simulink model "AdaptiveCruiseControl_HapticInterface"  (R2022b)
settings: Solver=FixedStepDiscrete  StartTime=0.0  StopTime=10.0  FixedStep=0.0005  RelTol=1e-3  EnableMultiTasking=on
InitFcn:
  | mbd_s32k_consistency_checks(bdroot(gcs));
values from neighbouring files (symbols this model uses):
  Ak = 100    [parameters_template.m]
  b = 100    [parameters_template.m]
  base_ids = [10, 0, 0, 0, 0, 0]    [parameters_template.m]
  dT = 0.01    [parameters_template.m]
  H = 20    [parameters_template.m]
  Kd = 0.0358    [parameters_template.m]
  Kdm = 137.4    [parameters_template.m]
  Kp = 0.256    [parameters_template.m]
  Kpm = 573.45    [parameters_template.m]
  L1 = 1.6    [parameters_template.m]
  L2 = 0.8    [parameters_template.m]
  m = 2000    [parameters_template.m]
  n_desired = 0    [parameters_template.m]
  pot_gain = 0.8    [parameters_template.m]
  pot_offset = 512    [parameters_template.m]
  R = 1/5    (= 0.2)    [parameters_template.m]
  V_Ki = 50    [parameters_template.m]
  V_Kp = 5000    [parameters_template.m]
undefined symbols (not defined in the file or in its folder): DiscIntNeverNeededParam, LQFP
libraries: mbd_s32k1xx_ec_toolbox x38, slrealtimeutilitieslib x15, Veh_Sim x9, simulink x3
(part 1 of 2)
settings Model: Creator=raoulkumar  LastModifiedBy=jyotshna
settings SolverCC: AlgebraicLoopSolver=TrustRegion  AutoInsertRateTranBlk=on
settings DataIOCC: ExternalInput=off  InitialState=off  LimitDataPoints=on  SaveOutput=off  SignalLogging=off  SaveTime=off  ReturnWorkspaceOutputs=off
settings OptimizationCC: DefaultParameterBehavior=Inlined  UseDivisionForNetSlopeComputation=on  UseFloatMulNetSlope=on  InlineInvariantSignals=on  EnhancedBackFolding=on  PassReuseOutputArgsAs=Individual arguments  ZeroExternalMemoryAtStartup=off  ZeroInternalMemoryAtStartup=off  NoFixptDivByZeroProtection=on  EfficientFloat2IntCast=on  OptimizeBlockOrder=speed  DifferentSizesBufferReuse=on  OptimizationCustomize=off  EfficientTunableParamExpr=on
settings DebuggingCC: InheritedTsInSrcMsg=none  SingleTaskRateTransMsg=error  ParameterTunabilityLossMsg=error  UnconnectedInputMsg=error  UnconnectedOutputMsg=error  UnconnectedLineMsg=error  AllowSymbolicDim=off  UnknownTsInhSupMsg=error  SFUnexpectedBacktrackingDiag=warning  SFNoUnconditionalDefaultTransitionDiag=warning  SFExecutionAtInitializationDiag=none  SFMachineParentedDataDiag=warning  ArithmeticOperatorsInVariantConditions=warning
settings HardwareCC: ProdBitPerPointer=32  ProdBitPerSizeT=32  ProdBitPerPtrDiffT=32  ProdLargestAtomicInteger=Long  ProdLargestAtomicFloat=Double  ProdWordSize=32  ProdHWDeviceType=ARM Compatible->ARM Cortex
settings ModelReferenceCC: EnableRefExpFcnMdlSchedulingChecks=on  PropagateSignalLabelsOutOfModel=off
settings SFSimCC: SimUseLocalCustomCode=off  MATLABDynamicMemAlloc=off  CustomCodeUndefinedFunction=UseInterfaceOnly
settings RTWCC: Description=Model Based Design Toolbox S32K1xx Code Generation Target  SystemTargetFile=mbd_s32k.tlc  MakeCommand=mbd_s32k_make_rtw COPY_MDLREF_INCLUDES=0  TemplateMakefile=mbd_s32k.tmf  GenerateReport=on  RTWUseLocalCustomCode=off  CustomHeaderCode=#include <math.h>  CustomSource=path_data.c;  IncludeHyperlinkInReport=on  LaunchReport=on  GenerateTraceInfo=on  GenerateTraceReport=on  GenerateTraceReportSl=on  GenerateTraceReportSf=on  GenerateTraceReportEml=on  GenerateCodeMetricsReport=on  DLArmComputeVersion=19.05
settings CodeAppCC: ForceParamTrailComments=on  IgnoreCustomStorageClasses=off  OperatorAnnotations=on  SimulinkDataObjDesc=on  SFDataObjDesc=on  CustomSymbolStrGlobalVar=rt$N$M  CustomSymbolStrType=$N$M  CustomSymbolStrFcn=$N$M$F  CustomSymbolStrMacro=$N$M  InsertBlockDesc=on
settings STFCustomTargetCC: TargetLangStandard=C99 (ISO)  MultiwordLength=256  CombineOutputUpdateFcns=on  ERTCustomFileBanners=on  SupportContinuousTime=off  SupportNonInlinedSFcns=off  RemoveResetFunc=on  MATLABClassNameForMDSCustomization=Simulink.SoftwareTarget.ERTCustomization  SystemTargetFile=mbd_s32k.tlc
settings ERTTargetCC: TargetLangStandard=C99 (ISO)  ParMdlRefBuildCompliant=off  CompOptLevelCompliant=off  ConcurrentExecutionCompliant=off  ModelStepFunctionPrototypeControlCompliant=off  CPPClassGenCompliant=off  UseToolchainInfoCompliant=off  InlinedParameterPlacement=NonHierarchical  ERTSrcFileBannerTemplate=mbd_ert_code_template.cgt  ERTHdrFileBannerTemplate=mbd_ert_code_template.cgt  ERTDataSrcFileTemplate=mbd_ert_code_template.cgt  ERTDataHdrFileTemplate=mbd_ert_code_template.cgt  ERTCustomFileTemplate=example_file_process.tlc
settings ConfigComp: CovMetricSettings=dw  CovSaveCumulativeToWorkspaceVar=on  CovSaveSingleToWorkspaceVar=on  CovExternalEMLEnable=off

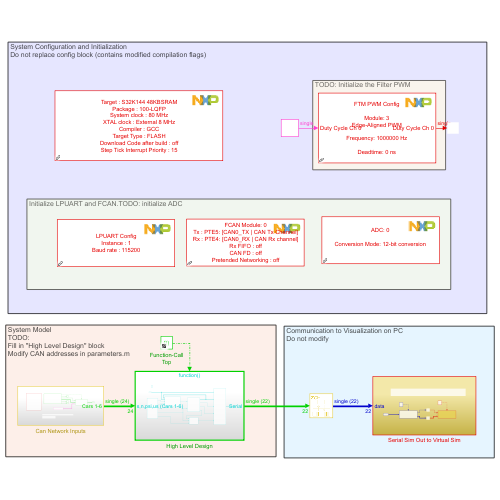
[thumbnail: Simulink's stored preview of the top-level diagram]
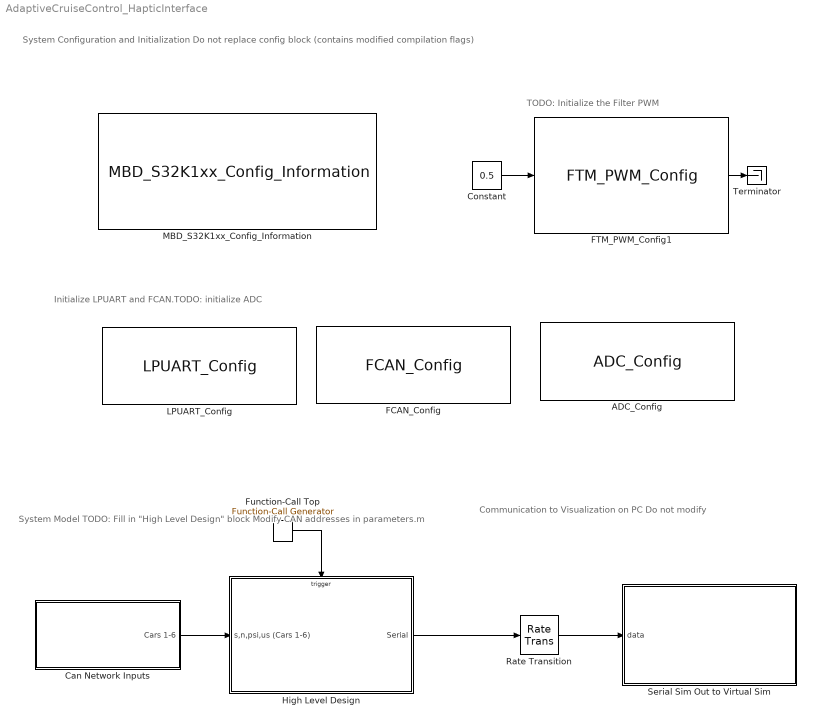
== system AdaptiveCruiseControl_HapticInterface ==
  note: TODO: Initialize the Filter PWM
  note: Communication to Visualization on PC
      | Do not modify
  note: Initialize LPUART and FCAN.TODO: initialize ADC
  note: System Configuration and Initialization
      | Do not replace config block (contains modified compilation flags)
  note: System Model
      | TODO:
      | Fill in "High Level Design" block
      | Modify CAN addresses in parameters.m
  ADC_Config : mbd_s32k1xx_ec_toolbox/Motor Control Blocks/ADC Blocks/ADC_Config  instance=0  mode=12-bit conversion  smplts=2  adiclk=alternate clock 1  adiv=input clock  show_adv_opts=off  pretrgsel=PDB pre-trigger  swpretrg=Disabled  adtrg=software  trgsel=TRGMUX output  refsel=Vrefh and Vrefl  supply_monitoring=off  acfe=off  acfgt=off  acren=off  cv1=0  cv2=0  adco=off  avge=off  avgs=4 samples
  Can Network Inputs : Subsystem
  Constant : Constant  Value=0.5  OutDataTypeStr=single
  FCAN_Config : mbd_s32k1xx_ec_toolbox/Communication Blocks/CAN Blocks/FCAN_Config  Priority=2  can_instance=0  can_mode=Normal mode  can_max_num_mb=32  can_rx=PTE4: [CAN0_RX | CAN Rx channel]  can_tx=PTE5: [CAN0_TX | CAN Tx Channel]  show_adv_opts=on  can_clk_src=Peripheral clock  can_clk_freq=80 MHz  bitrate_to_time_seg=on  bitrate=500  sample_point=80  real_bitrate=500  real_sample_point=80  prop_delay=250  bus_length=1  tq=200.0  time_quanta=10  can_presdiv=16  can_propseg=3  can_pseg1=4  can_pseg2=2  can_rjw=2  cbt_bitrate=2000  cbt_sample_point=80  cbt_real_bitrate=2000  cbt_real_sample_point=80  cbt_tq=25.0  cbt_time_quanta=40  can_cbt_presdiv=3  can_cbt_propseg=6  can_cbt_pseg1=7  can_cbt_pseg2=7  can_cbt_rjw=3  can_fd_enable=off  can_payload=8  tdc_enable=off  tdc_offset=20  can_rxfifo_enable=off  can_num_id_filters=8  can_fifo_id_format=A  can_fifo_id_filter={'0x0', '0x0', '0x0', '0x0', '0x0', '0x0', '0x0', '0x0'}  can_pn_enable=off  can_wakeup_match=off  can_wakeup_timeout=off  can_timeout_en=off  can_match_timeout=1  can_multiple_matches_en=off  can_num_matches=1  can_idfilter_extendedid=off  can_idfilter_remoteframe=off  can_idfilter_type=Match exact  can_idfilter_id1=0  can_idfilter_id2=0  can_payloadfilter_enable=off  can_payloadfilter_dlclow=0  can_payloadfilter_dlchigh=0  can_payloadfilter_type=Match exact  can_payloadfilter_payload1_b0=0  can_payloadfilter_payload1_b1=0  can_payloadfilter_payload1_b2=0  can_payloadfilter_payload1_b3=0  can_payloadfilter_payload1_b4=0  can_payloadfilter_payload1_b5=0  can_payloadfilter_payload1_b6=0  can_payloadfilter_payload1_b7=0  can_payloadfilter_payload2_b0=0  can_payloadfilter_payload2_b1=0  can_payloadfilter_payload2_b2=0  can_payloadfilter_payload2_b3=0  can_payloadfilter_payload2_b4=0  can_payloadfilter_payload2_b5=0  can_payloadfilter_payload2_b6=0  can_payloadfilter_payload2_b7=0
  FTM_PWM_Config1 : mbd_s32k1xx_ec_toolbox/Motor Control Blocks/FTM Blocks/FTM_PWM_Config  ftmModule=3  ftmMode=Edge-Aligned PWM  ftmSourceClock=80 MHz  swcontrol_enable=off  chan0En=on  chan0Type=Complementary  chan2En=off  chan2Type=Independent  chan4En=off  chan4Type=Independent  chan6En=off  chan6Type=Independent  ftmPwmUnits=Hz  outFrequency=1000000  ftmPeriod=80  ftmPrescaler=Divide by 1  deadtimeUnits=Nanoseconds  deadtimeNs=0  deadtimeTicks=0  deadtimePrescaler=Divide by 1  dutyCycleCh0=0.25  dutyCycleCh1=0.25  dutyCycleCh2=0.25  dutyCycleCh3=0.25  dutyCycleCh4=0.25  dutyCycleCh5=0.25  dutyCycleCh6=0.25  dutyCycleCh7=0.25  dutyCycleSim=on  startAfterInit=on  showAdvOpt=on  pinFtmCh0=PTB8: [FTM3_CH0 | FTM Channel]  pinFtmCh1=None  pinPolCh0=Active High  pinPolCh1=Active Low  outputComplem0=Main duplicated  outputLevel0=Low  outputLevel1=Low  pinFtmCh2=PTB10: [FTM3_CH2 | FTM Channel]  pinFtmCh3=None  pinPolCh2=Active Low  pinPolCh3=Active Low  outputComplem2=Main duplicated  outputLevel2=Low  outputLevel3=Low  pinFtmCh4=PTC10: [FTM3_CH4 | FTM Channel]  pinFtmCh5=None  pinPolCh4=Active Low  pinPolCh5=Active Low  outputComplem4=Main duplicated  outputLevel4=Low  outputLevel5=Low  pinFtmCh6=PTC12: [FTM3_CH6 | FTM Channel]  pinFtmCh7=None  pinPolCh6=Active Low  pinPolCh7=Active Low  outputComplem6=Main duplicated  outputLevel6=Low  outputLevel7=Low  initTrigger=off  chTrigger0=off  chTrigger1=off  chTrigger2=off  chTrigger3=off  chTrigger4=off  chTrigger5=off  chTrigger6=off  chTrigger7=off  mcuTargetUpdate=on  pwmSyncTrg=Software trigger  pwmSyncHwRouting=TRGMUX_FTM7  pwmSyncTrg0=off  pwmSyncTrg1=off  pwmSyncTrg2=off  pwmSyncAutoClear=on  pwmSyncMinLoad=on  pwmSyncMaxLoad=on  pwmSyncInvert=System Clock  pwmSyncOutControl=System Clock  pwmSyncOutMask=System Clock  pwmSyncCounterInitial=System Clock  pwmSyncPoints=Update now  reloadEnable=off  reloadPriority=15  reloadHalfCycle=off  reloadHCR=0  reloadFrequency=0  chnMatch0=off  chnMatch1=off  chnMatch2=off  chnMatch3=off  chnMatch4=off  chnMatch5=off  chnMatch6=off  chnMatch7=off  pwmFaultProtection=off  pwmFaultInterrupt=off  pwmFaultClearing=Fault control disabled  pwmFaultPinState=Safe Value  pwmFaultFilterValue=0  pwmFaultPriority=15  fault_disen_0=off  fault_filter_0=off  fault_polarity_0=Active High  fault_disen_1=off  fault_filter_1=off  fault_polarity_1=Active high  fault_disen_2=off  fault_filter_2=off  fault_polarity_2=Active high  fault_disen_3=off  fault_filter_3=off  fault_polarity_3=Active high  fault_pin_0=None  fault_pin_1=None  fault_pin_2=None  fault_pin_3=None
  Function-Call Top : simulink/Ports & Subsystems/Function-Call Generator  sample_time=dT  numberOfIterations=1  DisallowWideOutput=off
  High Level Design : Subsystem  TreatAsAtomicUnit=on
  LPUART_Config : mbd_s32k1xx_ec_toolbox/Communication Blocks/UART Blocks/LPUART_Config  Priority=2  instance=1  baudrate=115200  custom_baudrate=1000000  databits=8  parity=None  sbns=1  bothedge=rising edge  rxinv=off  txinv=off  show_adv_opts=on  brk13=10 - 13 bit times  lbkde=10 - 13 bit times  rx=PTC6: [LPUART1_RX | Receive]  tx=PTC7: [LPUART1_TX | Transmit]
  MBD_S32K1xx_Config_Information : mbd_s32k1xx_ec_toolbox/MBD_S32K1xx_Config_Information  mbdt_ver=0  disp_str=|  config_params=[]  mcu_target_name=S32K144  mcu_target_package=100-LQFP  mcu_target_sram_size=48KB  mcu_system_clock_freq=80  mcu_xtal_freq=External 8  mcu_steptick_timer=LPIT Channel 0  mcu_steptick_prio=15  ds_import_enable=on  target_compiler=GCC  target_memory=FLASH  gcc_target_compile_opts=-mthumb -mfloat-abi=hard -mfpu=fpv4-sp-d16 -O1 -g -gstrict-dwarf -DRT -DmwSize=size_t -include stdbool.h  gcc_target_assemble_opts=-mthumb -mfloat-abi=hard -mfpu=fpv4-sp-d16 -g  gcc_target_link_opts=-mthumb -mfloat-abi=hard -mfpu=fpv4-sp-d16  gcc_target_default_lcf=on  gcc_target_user_lcf=S32K144_48_flash.ld  ghs_target_compile_opts=-cpu=cortexm4f -thumb -fpu=vfpv4_d16 -fsingle -Ogeneral -Wundef -Wimplicit-int -Wshadow -Wtrigraphs --no_commons --gnu_asm -gnu99 -gdwarf-2 -G  ghs_target_assemble_opts=-cpu=cortexm4f -fpu=vfpv4_d16  ghs_target_link_opts=-cpu=cortexm4f -thumb -fpu=vfpv4_d16  ghs_target_default_lcf=on  ghs_target_user_lcf=S32K144_48_flash.ld  iar_target_compile_opts=--cpu=Cortex-M4F --thumb --fpu=VFPv4_sp -Ol -e --debug --dlib_config normal  iar_target_assemble_opts=--cpu Cortex-M4F --thumb --fpu VFPv4_sp  iar_target_link_opts=--no_exceptions --vfe --inline  iar_target_default_lcf=on  iar_target_user_lcf=S32K144_48_flash.icf  pil_download_enable=off  rbl_download_enable=off  rbl_start_delay=5000  rbl_download_interface=OpenSDA  rbl_restart_request=off  rbl_com_port=Custom  rbl_com_port_custom=COM1  pil_download_rate=57600  pil_download_rate_custom=115200  pil_opensda_drive=E: EVB-S32K144  pil_opensda_drive_custom=D  jtag_interface=OpenSDA Embedded Debug  jlink_default_path=on  jlink_user_path=C:\Program Files\SEGGER\JLink\  pil_uart_instance=1  pil_uart_rx=PTC6: [LPUART1_RX | Receive]  pil_uart_tx=PTC7: [LPUART1_TX | Transmit]  FTM_PWM_PcrCheckEnDis=on  FTM_Input_Edge_Inputs_PcrCheckEnDis=on  FTM_Dual_Edge_Inputs_PcrCheckEnDis=on  FTM_Quadrature_Inputs_PcrCheckEnDis=on  FTM_Hall_Sensor_Inputs_PcrCheckEnDis=on  LPTMR_PcrCheckEnDis=on  PIT_PcrCheckEnDis=on  RTC_PcrCheckEnDis=on  FlexCAN_PcrCheckEnDis=on  LIN_PcrCheckEnDis=on  FlexIO_PcrCheckEnDis=on  LPI2C_PcrCheckEnDis=on  LPSPI_PcrCheckEnDis=on  LPUART_PcrCheckEnDis=on  CMP_PcrCheckEnDis=on  GPIO_OutputPcrCheckEnDis=on  GPIO_InputPcrCheckEnDis=on  SBC_PcrCheckEnDis=on  BMS_PcrCheckEnDis=on  AMMCLIB_PcrCheckEnDis=on  FM_PcrCheckEnDis=on  Profile_PcrCheckEnDis=on  ConfigParams_PcrCheckEnDis=on  ModelRef_PcrCheckEnDis=on  PDB0_PcrCheckEnDis=on  CSEc_PcrCheckEnDis=on  eDMA_PcrCheckEnDis=on  FLASH_PcrCheckEnDis=on  ADC_PcrCheckEnDis=on  WDOG_PcrCheckEnDis=on
      | Target : S32K144-64KB_SRAM
      | Package : 100-pin
      | System clock : 80 MHz
      | XTAL clock : External 8 MHz
      | Compiler : IAR
      | Target Type : FLASH
      | Download Code after build : off
      | Step Tick Interrupt Priority : 15
  Rate Transition : RateTransition
  Serial Sim Out to Virtual Sim : Subsystem
  Terminator : Terminator
  wires:
  High Level Design/1(Serial) -> Rate Transition/1
  Function-Call Top/1 -> High Level Design/Trigger
  Rate Transition/1 -> Serial Sim Out to Virtual Sim/1(data)
  Can Network Inputs/1(Cars 1-6) -> High Level Design/1(s,n,psi,us (Cars 1-6))
  Constant/1 -> FTM_PWM_Config1/1
  FTM_PWM_Config1/1 -> Terminator/1

== system AdaptiveCruiseControl_HapticInterface/Can Network Inputs ==
  note: Do not modify anything here
      | Set base IDs in the parameters file
  note: These blocks may not display properly until CAN configuration has been comleted
  Array of 6 base IDs : Constant  Value=base_ids
  Can Message Mailbox Setup : Subsystem
  Extract CAN data : Subsystem
  FCAN_Isr : mbd_s32k1xx_ec_toolbox/Communication Blocks/CAN Blocks/FCAN_Isr  can_instance=0  can_event=Rx Complete
  Terminator1 : Terminator
  Terminator2 : Terminator
  Terminator3 : Terminator
  Cars 1-6 : Outport  VectorParamsAs1DForOutWhenUnconnected=off
  wires:
  FCAN_Isr/5 -> Terminator1/1
  Array of 6 base IDs/1 -> Extract CAN data/3(CAN Base IDs (Cars 1-6))
  FCAN_Isr/4 -> Extract CAN data/2(data)
  FCAN_Isr/6 -> Terminator3/1
  FCAN_Isr/1 -> Extract CAN data/Trigger
  Extract CAN data/1("s, n, psi, us (Cars 1-6)") -> Cars 1-6/1
  FCAN_Isr/2 -> Terminator2/1
  FCAN_Isr/3 -> Extract CAN data/1(ID)

== system AdaptiveCruiseControl_HapticInterface/High Level Design ==
  s,n,psi,us (Cars 1-6) : Inport
  function : TriggerPort  TriggerType=function-call  VariantControl=(inherit)
  ACC : Subsystem
  Auto Steer : Subsystem
  Inputs : Subsystem
  Outputs : Subsystem
  Vehicle Dynamics : Subsystem
  Serial : Outport  VectorParamsAs1DForOutWhenUnconnected=off
  wires:
  Outputs/1("x, y, pxi (Cars 1-6)") -> Serial/1
  Inputs/4(Steering Angle (delta)) -> Vehicle Dynamics/2(delta), Auto Steer/2(delta)
  Vehicle Dynamics/3(self-align torque) -> Outputs/4(Self-Aligning Torque)
  Vehicle Dynamics/2(u (this car)) -> Outputs/3(u (This car))
  Vehicle Dynamics/1(s,n,psi,u_s (this car)) -> ACC/1(s,n,psi,us (This car)), Outputs/2("s, n, psi, us (This Car)")
  s,n,psi,us (Cars 1-6)/1 -> ACC/2(s,n,psi,us (Cars 1-6)), Outputs/1("s, n, psi, us (Cars 1-6)")
  Inputs/1(ACC_enable) -> ACC/3(ACC_EN)
  Inputs/2(Cruise Control Speed) -> ACC/4(Cruise Speed)
  Inputs/3(Throttle (Fd)) -> ACC/5(Throttle)
  ACC/1(F_d) -> Vehicle Dynamics/1(F_d)
  Auto Steer/1(Auto Torque) -> Outputs/5(Auto Torque)
  Vehicle Dynamics/4(n) -> Auto Steer/1(n)
  Inputs/5(Automatic Steering Enable) -> Auto Steer/3(AS_EN)

== system AdaptiveCruiseControl_HapticInterface/Serial Sim Out to Virtual Sim ==
  note: UART transmission is non-blocking.
      | We must wait for transmission to complete before sending the next byte.
      | Could use LPUART interrupts block or just periodcally transmit to allow time for buffer to clear
  data : Inport
  Function-Call Generator1 : simulink/Ports & Subsystems/Function-Call Generator  sample_time=0.05  numberOfIterations=1  DisallowWideOutput=off
  Function-Call Generator2 : simulink/Ports & Subsystems/Function-Call Generator  sample_time=0.05 / 100  numberOfIterations=1  DisallowWideOutput=off
  RT : RateTransition  OutPortSampleTimeOpt=Inherit  OutPortSampleTime=0.0005
  RT1 : RateTransition  OutPortSampleTimeOpt=Inherit  OutPortSampleTime=0.0005
  Serial : Subsystem  TreatAsAtomicUnit=on
  UART Iteration : Subsystem
  wires:
  Serial/1(reset) -> RT/1
  Serial/2(data_out) -> RT1/1
  data/1 -> Serial/1(data)
  Function-Call Generator1/1 -> Serial/Trigger
  RT/1 -> UART Iteration/1(reset)
  Function-Call Generator2/1 -> UART Iteration/Trigger
  RT1/1 -> UART Iteration/2(data)

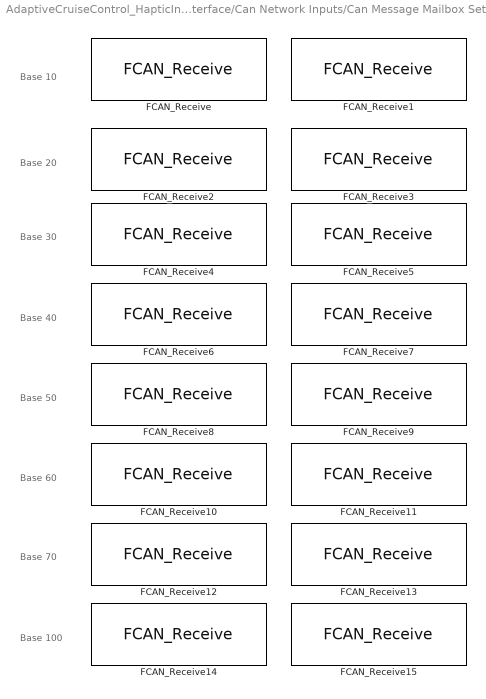
== system AdaptiveCruiseControl_HapticInterface/Can Network Inputs/Can Message Mailbox Setup ==
  note: Base 10
  note: Base 20
  note: Base 30
  note: Base 40
  note: Base 50
  note: Base 60
  note: Base 70
  note: Base 100
  FCAN_Receive : mbd_s32k1xx_ec_toolbox/Communication Blocks/CAN Blocks/FCAN_Receive  can_instance=0  can_mode=Non-blocking  can_timeout_ms=0  can_mb_idx=16  can_mb_init=Once  show_id_input=off  can_extended_id=off  can_is_remote=off  can_id=0F  can_msg_mask=0  show_adv_opts=on  can_use_rxfifo=off  can_fd_enable=off
  FCAN_Receive1 : mbd_s32k1xx_ec_toolbox/Communication Blocks/CAN Blocks/FCAN_Receive  can_instance=0  can_mode=Non-blocking  can_timeout_ms=0  can_mb_idx=17  can_mb_init=Once  show_id_input=off  can_extended_id=off  can_is_remote=off  can_id=10  can_msg_mask=0  show_adv_opts=on  can_use_rxfifo=off  can_fd_enable=off
  FCAN_Receive10 : mbd_s32k1xx_ec_toolbox/Communication Blocks/CAN Blocks/FCAN_Receive  can_instance=0  can_mode=Non-blocking  can_timeout_ms=0  can_mb_idx=12  can_mb_init=Once  show_id_input=off  can_extended_id=off  can_is_remote=off  can_id=41  can_msg_mask=0  show_adv_opts=on  can_use_rxfifo=off  can_fd_enable=off
  FCAN_Receive11 : mbd_s32k1xx_ec_toolbox/Communication Blocks/CAN Blocks/FCAN_Receive  can_instance=0  can_mode=Non-blocking  can_timeout_ms=0  can_mb_idx=13  can_mb_init=Once  show_id_input=off  can_extended_id=off  can_is_remote=off  can_id=42  can_msg_mask=0  show_adv_opts=on  can_use_rxfifo=off  can_fd_enable=off
  FCAN_Receive12 : mbd_s32k1xx_ec_toolbox/Communication Blocks/CAN Blocks/FCAN_Receive  can_instance=0  can_mode=Non-blocking  can_timeout_ms=0  can_mb_idx=2  can_mb_init=Once  show_id_input=off  can_extended_id=off  can_is_remote=off  can_id=4b  can_msg_mask=0  show_adv_opts=on  can_use_rxfifo=off  can_fd_enable=off
  FCAN_Receive13 : mbd_s32k1xx_ec_toolbox/Communication Blocks/CAN Blocks/FCAN_Receive  can_instance=0  can_mode=Non-blocking  can_timeout_ms=0  can_mb_idx=3  can_mb_init=Once  show_id_input=off  can_extended_id=off  can_is_remote=off  can_id=4c  can_msg_mask=0  show_adv_opts=on  can_use_rxfifo=off  can_fd_enable=off
  FCAN_Receive14 : mbd_s32k1xx_ec_toolbox/Communication Blocks/CAN Blocks/FCAN_Receive  can_instance=0  can_mode=Non-blocking  can_timeout_ms=0  can_mb_idx=14  can_mb_init=Once  show_id_input=off  can_extended_id=off  can_is_remote=off  can_id=69  can_msg_mask=0  show_adv_opts=on  can_use_rxfifo=off  can_fd_enable=off
  FCAN_Receive15 : mbd_s32k1xx_ec_toolbox/Communication Blocks/CAN Blocks/FCAN_Receive  can_instance=0  can_mode=Non-blocking  can_timeout_ms=0  can_mb_idx=15  can_mb_init=Once  show_id_input=off  can_extended_id=off  can_is_remote=off  can_id=6a  can_msg_mask=0  show_adv_opts=on  can_use_rxfifo=off  can_fd_enable=off
  FCAN_Receive2 : mbd_s32k1xx_ec_toolbox/Communication Blocks/CAN Blocks/FCAN_Receive  can_instance=0  can_mode=Non-blocking  can_timeout_ms=0  can_mb_idx=4  can_mb_init=Once  show_id_input=off  can_extended_id=off  can_is_remote=off  can_id=19  can_msg_mask=0  show_adv_opts=on  can_use_rxfifo=off  can_fd_enable=off
  FCAN_Receive3 : mbd_s32k1xx_ec_toolbox/Communication Blocks/CAN Blocks/FCAN_Receive  can_instance=0  can_mode=Non-blocking  can_timeout_ms=0  can_mb_idx=5  can_mb_init=Once  show_id_input=off  can_extended_id=off  can_is_remote=off  can_id=1a  can_msg_mask=0  show_adv_opts=on  can_use_rxfifo=off  can_fd_enable=off
  FCAN_Receive4 : mbd_s32k1xx_ec_toolbox/Communication Blocks/CAN Blocks/FCAN_Receive  can_instance=0  can_mode=Non-blocking  can_timeout_ms=0  can_mb_idx=6  can_mb_init=Once  show_id_input=off  can_extended_id=off  can_is_remote=off  can_id=23  can_msg_mask=0  show_adv_opts=on  can_use_rxfifo=off  can_fd_enable=off
  FCAN_Receive5 : mbd_s32k1xx_ec_toolbox/Communication Blocks/CAN Blocks/FCAN_Receive  can_instance=0  can_mode=Non-blocking  can_timeout_ms=0  can_mb_idx=7  can_mb_init=Once  show_id_input=off  can_extended_id=off  can_is_remote=off  can_id=24  can_msg_mask=0  show_adv_opts=on  can_use_rxfifo=off  can_fd_enable=off
  FCAN_Receive6 : mbd_s32k1xx_ec_toolbox/Communication Blocks/CAN Blocks/FCAN_Receive  can_instance=0  can_mode=Non-blocking  can_timeout_ms=0  can_mb_idx=8  can_mb_init=Once  show_id_input=off  can_extended_id=off  can_is_remote=off  can_id=2d  can_msg_mask=0  show_adv_opts=on  can_use_rxfifo=off  can_fd_enable=off
  FCAN_Receive7 : mbd_s32k1xx_ec_toolbox/Communication Blocks/CAN Blocks/FCAN_Receive  can_instance=0  can_mode=Non-blocking  can_timeout_ms=0  can_mb_idx=9  can_mb_init=Once  show_id_input=off  can_extended_id=off  can_is_remote=off  can_id=2e  can_msg_mask=0  show_adv_opts=on  can_use_rxfifo=off  can_fd_enable=off
  FCAN_Receive8 : mbd_s32k1xx_ec_toolbox/Communication Blocks/CAN Blocks/FCAN_Receive  can_instance=0  can_mode=Non-blocking  can_timeout_ms=0  can_mb_idx=10  can_mb_init=Once  show_id_input=off  can_extended_id=off  can_is_remote=off  can_id=37  can_msg_mask=0  show_adv_opts=on  can_use_rxfifo=off  can_fd_enable=off
  FCAN_Receive9 : mbd_s32k1xx_ec_toolbox/Communication Blocks/CAN Blocks/FCAN_Receive  can_instance=0  can_mode=Non-blocking  can_timeout_ms=0  can_mb_idx=11  can_mb_init=Once  show_id_input=off  can_extended_id=off  can_is_remote=off  can_id=38  can_msg_mask=0  show_adv_opts=on  can_use_rxfifo=off  can_fd_enable=off

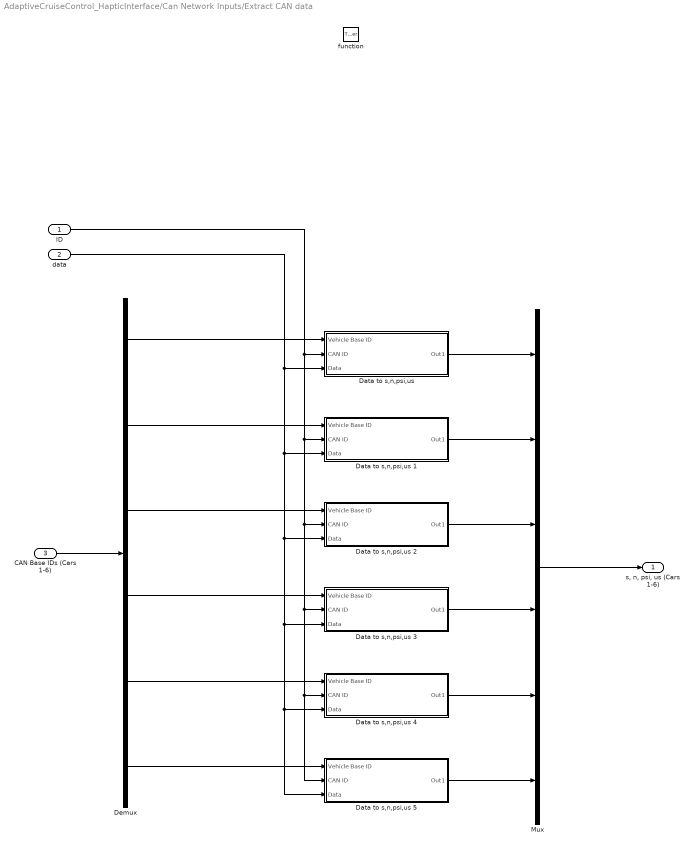
== system AdaptiveCruiseControl_HapticInterface/Can Network Inputs/Extract CAN data ==
  ID : Inport
  data : Inport  Port=2
  CAN Base IDs (Cars 1-6) : Inport  Port=3
  function : TriggerPort  TriggerType=function-call  VariantControl=Variant
  "Data to s,n,psi,us " : Subsystem
  Data to s,n,psi,us 1 : Subsystem
  Data to s,n,psi,us 2 : Subsystem
  Data to s,n,psi,us 3 : Subsystem
  Data to s,n,psi,us 4 : Subsystem
  Data to s,n,psi,us 5 : Subsystem
  Demux : Demux  Outputs=6
  Mux : Mux  Inputs=6
  "s, n, psi, us (Cars 1-6)" : Outport  VectorParamsAs1DForOutWhenUnconnected=off
  wires:
  Mux/1 -> "s, n, psi, us (Cars 1-6)"/1
  ID/1 -> Data to s,n,psi,us 5/2(CAN ID), Data to s,n,psi,us 4/2(CAN ID), Data to s,n,psi,us 3/2(CAN ID), Data to s,n,psi,us 2/2(CAN ID), Data to s,n,psi,us 1/2(CAN ID), "Data to s,n,psi,us "/2(CAN ID)
  "Data to s,n,psi,us "/1(Out1) -> Mux/1
  Data to s,n,psi,us 1/1(Out1) -> Mux/2
  Data to s,n,psi,us 2/1(Out1) -> Mux/3
  Data to s,n,psi,us 3/1(Out1) -> Mux/4
  Data to s,n,psi,us 4/1(Out1) -> Mux/5
  Data to s,n,psi,us 5/1(Out1) -> Mux/6
  data/1 -> Data to s,n,psi,us 5/3(Data), Data to s,n,psi,us 4/3(Data), Data to s,n,psi,us 3/3(Data), Data to s,n,psi,us 2/3(Data), Data to s,n,psi,us 1/3(Data), "Data to s,n,psi,us "/3(Data)
  Demux/1 -> "Data to s,n,psi,us "/1(Vehicle Base ID)
  Demux/2 -> Data to s,n,psi,us 1/1(Vehicle Base ID)
  Demux/3 -> Data to s,n,psi,us 2/1(Vehicle Base ID)
  Demux/4 -> Data to s,n,psi,us 3/1(Vehicle Base ID)
  Demux/5 -> Data to s,n,psi,us 4/1(Vehicle Base ID)
  Demux/6 -> Data to s,n,psi,us 5/1(Vehicle Base ID)
  CAN Base IDs (Cars 1-6)/1 -> Demux/1

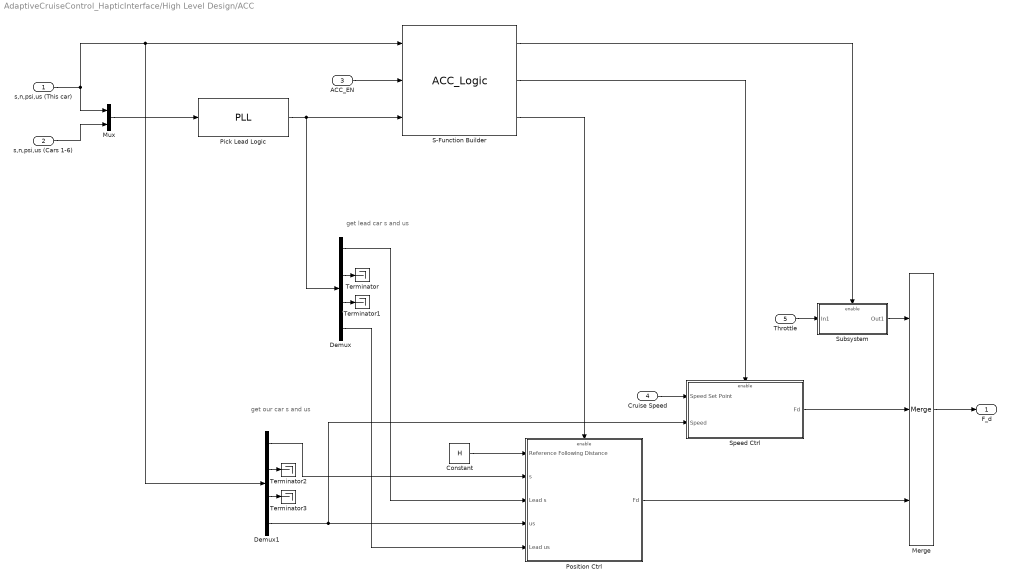
== system AdaptiveCruiseControl_HapticInterface/High Level Design/ACC ==
  note: get our car s and us
  note: get lead car s and us
  s,n,psi,us (This car) : Inport
  s,n,psi,us (Cars 1-6) : Inport  Port=2
  ACC_EN : Inport  Port=3
  Cruise Speed : Inport  Port=4
  Throttle : Inport  Port=5
  Constant : Constant  Value=H
  Demux : Demux
  Demux1 : Demux
  Merge : Merge  Inputs=3
  Mux : Mux  Inputs=2
  Pick Lead Logic : S-Function  FunctionName=PLL  SFunctionModules=PLL_wrapper.c  SFunctionDeploymentMode=off  EnableBusSupport=off  mask(S-Function Builder){}
      mask help: Simulink:masks:SFunctionBuilder_MD
      mask init:
      | val = [[.9  0.75 0.75 1 1 .9 .9 1]',[1 1 0.75 0.75 .9 .9 1 .9]'];try , sys = get_param(gcb,'SfunBuilderFcnName');if isempty(sys), sys = get_param(gcb,'FunctionName'); end,catch, sys = get_param(gcb,'FunctionName'); end
      settings: CopyFcn=set_param(gcbh,'LinkStatus','none')  OpenFcn=sfunctionwizard(gcbh)
      mask Display:
      | plot(val(:,1),val(:,2))
      | disp(sys)
      | port_label('input',1,'cars')
      | port_label('output',1,'lead')
  Position Ctrl : Subsystem  TreatAsAtomicUnit=on
  S-Function Builder : S-Function  FunctionName=ACC_Logic  Parameters=single(H)  SFunctionModules=ACC_Logic_wrapper.c  SFunctionDeploymentMode=off  EnableBusSupport=off  mask(S-Function Builder){}
      mask help: Simulink:masks:SFunctionBuilder_MD
      mask init: same as AdaptiveCruiseControl_HapticInterface/High Level Design/ACC/Pick Lead Logic
      settings: CopyFcn=set_param(gcbh,'LinkStatus','none')  OpenFcn=sfunctionwizard(gcbh)
      mask Display:
      | plot(val(:,1),val(:,2))
      | disp(sys)
      | port_label('input',1,'our_car')
      | port_label('input',2,'ACC_EN')
      | port_label('input',3,'lead_car')
      | port_label('output',1,'MAN_EN')
      | port_label('output',2,'VEL_EN')
      | port_label('output',3,'POS_EN')
  Speed Ctrl : Subsystem  TreatAsAtomicUnit=on
  Subsystem : Subsystem
  Terminator{,1..3} (4 alike) : Terminator
  F_d : Outport
  wires:
  S-Function Builder/1 -> Subsystem/Enable
  Demux/1 -> Position Ctrl/3(Lead s)
  Demux/3 -> Terminator1/1
  Demux1/2 -> Terminator2/1
  s,n,psi,us (This car)/1 -> Mux/1, Demux1/1, S-Function Builder/1
  s,n,psi,us (Cars 1-6)/1 -> Mux/2
  Demux1/1 -> Position Ctrl/2(s)
  Mux/1 -> Pick Lead Logic/1
  ACC_EN/1 -> S-Function Builder/2
  Position Ctrl/1(Fd) -> Merge/3
  Demux/4 -> Position Ctrl/5(Lead us)
  S-Function Builder/3 -> Position Ctrl/Enable
  Subsystem/1(Out1) -> Merge/1
  Pick Lead Logic/1 -> Demux/1, S-Function Builder/3
  Constant/1 -> Position Ctrl/1(Reference Following Distance)
  Throttle/1 -> Subsystem/1(In1)
  Demux/2 -> Terminator/1
  Demux1/4 -> Speed Ctrl/2(Speed), Position Ctrl/4(us)
  Demux1/3 -> Terminator3/1
  Cruise Speed/1 -> Speed Ctrl/1(Speed Set Point)
  Speed Ctrl/1(Fd) -> Merge/2
  S-Function Builder/2 -> Speed Ctrl/Enable
  Merge/1 -> F_d/1

== system AdaptiveCruiseControl_HapticInterface/High Level Design/Auto Steer ==
  n : Inport
  delta : Inport  Port=2
  AS_EN : Inport  Port=3
  S-Function Builder1 : S-Function  Commented=on  FunctionName=auto_steer  Parameters=single(n_desired),single(Kp),single(Kd),single(Kpm),single(Kdm)  SFunctionModules=auto_steer_wrapper.c  SFunctionDeploymentMode=off  EnableBusSupport=off  mask(S-Function Builder){}
      mask help: Simulink:masks:SFunctionBuilder_MD
      mask init: same as AdaptiveCruiseControl_HapticInterface/High Level Design/ACC/Pick Lead Logic
      settings: CopyFcn=set_param(gcbh,'LinkStatus','none')  OpenFcn=sfunctionwizard(gcbh)
      mask Display:
      | plot(val(:,1),val(:,2))
      | disp(sys)
      | port_label('input',1,'n')
      | port_label('input',2,'delta')
      | port_label('input',3,'AS_EN')
      | port_label('output',1,'t_auto')
  Subsystem1 : Subsystem
  Auto Torque : Outport
  wires:
  n/1 -> Subsystem1/1(n)
  delta/1 -> Subsystem1/2(delta)
  AS_EN/1 -> Subsystem1/3(AS_EN)
  Subsystem1/1(Auto-steer torque) -> Auto Torque/1

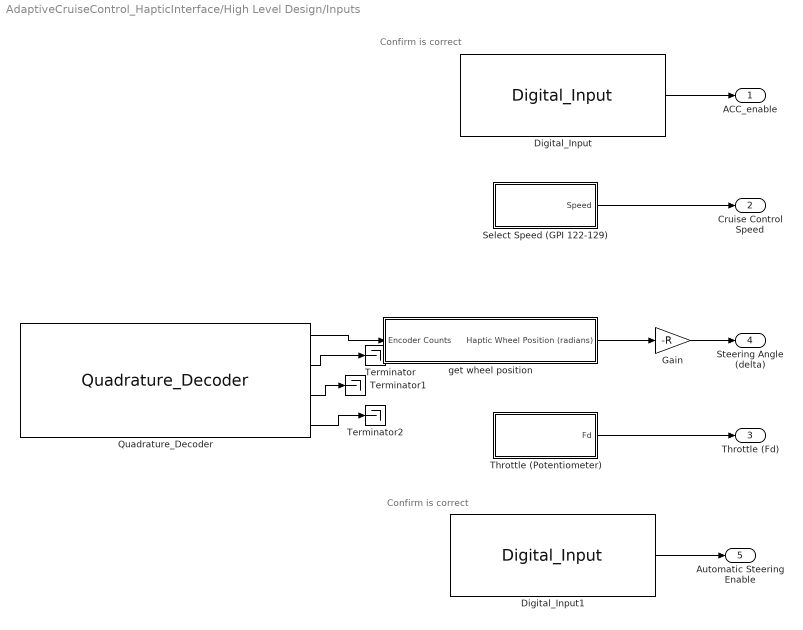
== system AdaptiveCruiseControl_HapticInterface/High Level Design/Inputs ==
  note: Confirm is correct
  note: Confirm is correct
  Digital_Input : mbd_s32k1xx_ec_toolbox/GPIO Blocks/Digital_Input  gpio_pin=PTE14: [PTE14 | Port E I/O]  pull_resistor=None  passive_filter=off
  Digital_Input1 : mbd_s32k1xx_ec_toolbox/GPIO Blocks/Digital_Input  gpio_pin=PTE15: [PTE15 | Port E I/O]  pull_resistor=None  passive_filter=off
  Gain : Gain  Gain=-R  OutDataTypeStr=single
  Quadrature_Decoder : mbd_s32k1xx_ec_toolbox/Motor Control Blocks/FTM Blocks/Quadrature_Decoder  Priority=1  ftmModule=2  ec_mode=Phase A and Phase B  prescaler=1  cntin=0  mod=65535  phA_filtr_en=off  phA_filter=0  phA_pin=PTA13: [FTM2_QD_PHA | FTM quadrature Decode PhaseA]  polA=Normal  phB_filtr_en=off  phB_filter=0  phB_pin=PTA12: [FTM2_QD_PHB | FTM quadrature Decode PhaseB]  polB=Normal
  Select Speed (GPI 122-129) : Subsystem
  Terminator : Terminator
  Terminator1 : Terminator
  Terminator2 : Terminator
  Throttle (Potentiometer) : Subsystem
  get wheel position : Subsystem
  ACC_enable : Outport  VectorParamsAs1DForOutWhenUnconnected=off
  Cruise Control Speed : Outport  Port=2  VectorParamsAs1DForOutWhenUnconnected=off
  Throttle (Fd) : Outport  Port=3  VectorParamsAs1DForOutWhenUnconnected=off
  Steering Angle (delta) : Outport  Port=4  VectorParamsAs1DForOutWhenUnconnected=off
  Automatic Steering Enable : Outport  Port=5  VectorParamsAs1DForOutWhenUnconnected=off
  wires:
  Select Speed (GPI 122-129)/1(Speed) -> Cruise Control Speed/1
  get wheel position/1(Haptic Wheel Position (radians)) -> Gain/1
  Gain/1 -> Steering Angle (delta)/1
  Throttle (Potentiometer)/1(Fd) -> Throttle (Fd)/1
  Digital_Input1/1 -> Automatic Steering Enable/1
  Digital_Input/1 -> ACC_enable/1
  Quadrature_Decoder/4 -> Terminator2/1
  Quadrature_Decoder/1 -> get wheel position/1(Encoder Counts)
  Quadrature_Decoder/2 -> Terminator/1
  Quadrature_Decoder/3 -> Terminator1/1

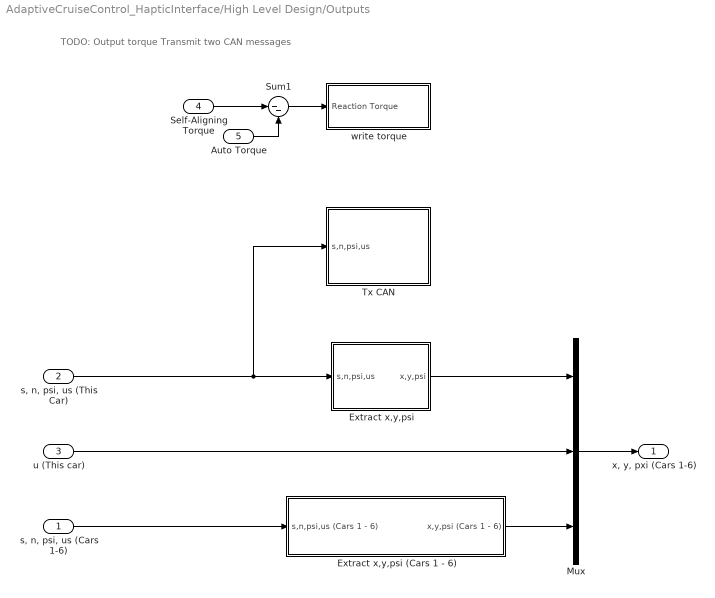
== system AdaptiveCruiseControl_HapticInterface/High Level Design/Outputs ==
  note: TODO:
      | Output torque
      | Transmit two CAN messages
  "s, n, psi, us (Cars 1-6)" : Inport
  "s, n, psi, us (This Car)" : Inport  Port=2
  u (This car) : Inport  Port=3
  Self-Aligning Torque : Inport  Port=4
  Auto Torque : Inport  Port=5
  Extract x,y,psi : Subsystem
  Extract x,y,psi (Cars 1 - 6) : Subsystem
  Mux : Mux  Inputs=3
  Sum1 : Sum  Inputs=|--
  Tx CAN : Subsystem
  write torque : Subsystem
  "x, y, pxi (Cars 1-6)" : Outport  VectorParamsAs1DForOutWhenUnconnected=off
  wires:
  Self-Aligning Torque/1 -> Sum1/1
  Auto Torque/1 -> Sum1/2
  Sum1/1 -> write torque/1(Reaction Torque)
  "s, n, psi, us (Cars 1-6)"/1 -> Extract x,y,psi (Cars 1 - 6)/1(s,n,psi,us (Cars 1 - 6))
  "s, n, psi, us (This Car)"/1 -> Tx CAN/1(s,n,psi,us), Extract x,y,psi/1(s,n,psi,us)
  Extract x,y,psi/1(x,y,psi) -> Mux/1
  Mux/1 -> "x, y, pxi (Cars 1-6)"/1
  u (This car)/1 -> Mux/2
  Extract x,y,psi (Cars 1 - 6)/1(x,y,psi (Cars 1 - 6)) -> Mux/3

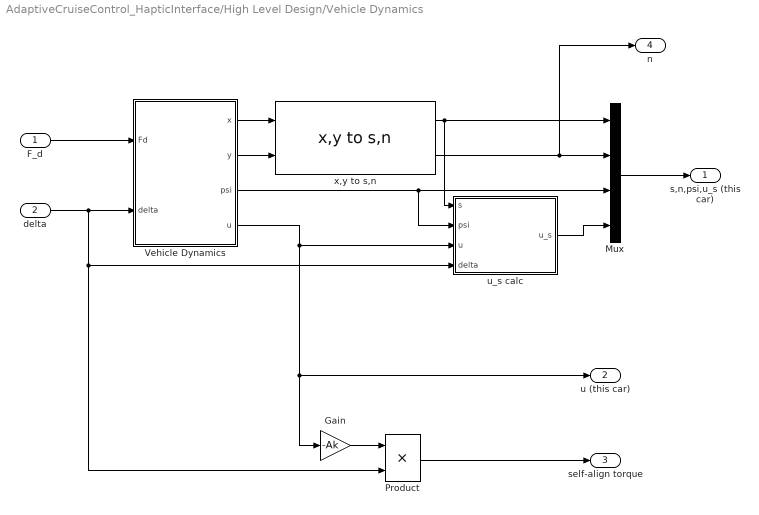
== system AdaptiveCruiseControl_HapticInterface/High Level Design/Vehicle Dynamics ==
  F_d : Inport
  delta : Inport  Port=2
  Gain : Gain  Gain=-Ak
  Mux : Mux
  Product : Product
  Vehicle Dynamics : Subsystem
  u_s calc : Subsystem
  x,y to s,n : Veh_Sim/x,y to s,n  SystemSampleTime=-1  VariantActivationTime=update diagram  Latency=0  AutoFrameSizeCalculation=off
  s,n,psi,u_s (this car) : Outport
  u (this car) : Outport  Port=2
  self-align torque : Outport  Port=3
  n : Outport  Port=4
  wires:
  F_d/1 -> Vehicle Dynamics/1(Fd)
  delta/1 -> Vehicle Dynamics/2(delta), Product/2, u_s calc/4(delta)
  Vehicle Dynamics/1(x) -> x,y to s,n/1
  Vehicle Dynamics/2(y) -> x,y to s,n/2
  Vehicle Dynamics/4(u) -> u_s calc/3(u), Gain/1, u (this car)/1
  Gain/1 -> Product/1
  Product/1 -> self-align torque/1
  x,y to s,n/1 -> Mux/1, u_s calc/1(s)
  x,y to s,n/2 -> Mux/2, n/1
  Vehicle Dynamics/3(psi) -> Mux/3, u_s calc/2(psi)
  Mux/1 -> s,n,psi,u_s (this car)/1
  u_s calc/1(u_s) -> Mux/4

== system AdaptiveCruiseControl_HapticInterface/Serial Sim Out to Virtual Sim/Serial ==
  data : Inport
  Trigger : TriggerPort  TriggerType=function-call  VariantControl=(inherit)
  "Byte Packing " : slrealtimeutilitieslib/Byte Packing  MaskPackedDataType=uint8  MaskUnpackedDataTypes={'single'}  MaskAlignment=1
  Constant2 : Constant  Value=uint8('s')  OutDataTypeStr=uint8
  Constant3 : Constant  Value=uint8('e')  OutDataTypeStr=uint8
  Delay : Delay  DelayLength=1
  Mux : Mux  Inputs=3
  NOT : Logic  Operator=NOT  IconShape=distinctive  AllPortsSameDT=off  OutDataTypeStr=boolean
  reset : Outport  VectorParamsAs1DForOutWhenUnconnected=off
  data_out : Outport  Port=2  VectorParamsAs1DForOutWhenUnconnected=off
  wires:
  Constant2/1 -> Mux/1
  Constant3/1 -> Mux/3
  Delay/1 -> NOT/1
  NOT/1 -> reset/1, Delay/1
  Mux/1 -> data_out/1
  "Byte Packing "/1 -> Mux/2
  data/1 -> "Byte Packing "/1

== system AdaptiveCruiseControl_HapticInterface/Serial Sim Out to Virtual Sim/UART Iteration ==
  reset : Inport
  data : Inport  Port=2
  Trigger : TriggerPort  TriggerType=function-call  VariantControl=(inherit)
  Index Vector : MultiPortSwitch  Inputs=1  SaturateOnIntegerOverflow=off  InputSameDT=off
  LPUART_Transmit : mbd_s32k1xx_ec_toolbox/Communication Blocks/UART Blocks/LPUART_Transmit  instance=1  transmit_mode=Non-blocking  timeout=500  number=off
  Resettable Subsystem : Subsystem  TreatAsAtomicUnit=on
  wires:
  data/1 -> Index Vector/2
  Index Vector/1 -> LPUART_Transmit/1
  reset/1 -> Resettable Subsystem/Reset
  Resettable Subsystem/1(Out1) -> Index Vector/1

== system AdaptiveCruiseControl_HapticInterface/Can Network Inputs/Extract CAN data/Data to s,n,psi,us  ==
  Vehicle Base ID : Inport
  CAN ID : Inport  Port=2
  Data : Inport  Port=3
  If : If  IfExpression=u1 == 5  ElseIfExpressions=u1 == 6  ShowElse=off
  Mux3 : Mux
  Subtract : Sum  Inputs=+-
  Switch Case Action Subsystem2 : Subsystem  TreatAsAtomicUnit=on
  Switch Case Action Subsystem3 : Subsystem  TreatAsAtomicUnit=on
  Out1 : Outport  VectorParamsAs1DForOutWhenUnconnected=off
  wires:
  If/2 -> Switch Case Action Subsystem3/Action
  Switch Case Action Subsystem2/2(n) -> Mux3/2
  Mux3/1 -> Out1/1
  Switch Case Action Subsystem3/2(us) -> Mux3/4
  Switch Case Action Subsystem3/1(psi) -> Mux3/3
  Data/1 -> Switch Case Action Subsystem2/1(s,n), Switch Case Action Subsystem3/1(psi,us)
  Switch Case Action Subsystem2/1(s) -> Mux3/1
  CAN ID/1 -> Subtract/1
  Vehicle Base ID/1 -> Subtract/2
  Subtract/1 -> If/1
  If/1 -> Switch Case Action Subsystem2/Action

== system AdaptiveCruiseControl_HapticInterface/Can Network Inputs/Extract CAN data/Data to s,n,psi,us 1 ==
  Vehicle Base ID : Inport
  CAN ID : Inport  Port=2
  Data : Inport  Port=3
  If : If  IfExpression=u1 == 5  ElseIfExpressions=u1 == 6  ShowElse=off
  Mux3 : Mux
  Subtract : Sum  Inputs=+-
  Switch Case Action Subsystem2 : Subsystem  TreatAsAtomicUnit=on
  Switch Case Action Subsystem3 : Subsystem  TreatAsAtomicUnit=on
  Out1 : Outport  VectorParamsAs1DForOutWhenUnconnected=off
  wires:
  If/2 -> Switch Case Action Subsystem3/Action
  Switch Case Action Subsystem2/2(n) -> Mux3/2
  Mux3/1 -> Out1/1
  Switch Case Action Subsystem3/2(us) -> Mux3/4
  Switch Case Action Subsystem3/1(psi) -> Mux3/3
  Data/1 -> Switch Case Action Subsystem2/1(s,n), Switch Case Action Subsystem3/1(psi,us)
  Switch Case Action Subsystem2/1(s) -> Mux3/1
  CAN ID/1 -> Subtract/1
  Vehicle Base ID/1 -> Subtract/2
  Subtract/1 -> If/1
  If/1 -> Switch Case Action Subsystem2/Action

== system AdaptiveCruiseControl_HapticInterface/Can Network Inputs/Extract CAN data/Data to s,n,psi,us 2 ==
  Vehicle Base ID : Inport
  CAN ID : Inport  Port=2
  Data : Inport  Port=3
  If : If  IfExpression=u1 == 5  ElseIfExpressions=u1 == 6  ShowElse=off
  Mux3 : Mux
  Subtract : Sum  Inputs=+-
  Switch Case Action Subsystem2 : Subsystem  TreatAsAtomicUnit=on
  Switch Case Action Subsystem3 : Subsystem  TreatAsAtomicUnit=on
  Out1 : Outport  VectorParamsAs1DForOutWhenUnconnected=off
  wires:
  If/2 -> Switch Case Action Subsystem3/Action
  Switch Case Action Subsystem2/2(n) -> Mux3/2
  Mux3/1 -> Out1/1
  Switch Case Action Subsystem3/2(us) -> Mux3/4
  Switch Case Action Subsystem3/1(psi) -> Mux3/3
  Data/1 -> Switch Case Action Subsystem2/1(s,n), Switch Case Action Subsystem3/1(psi,us)
  Switch Case Action Subsystem2/1(s) -> Mux3/1
  CAN ID/1 -> Subtract/1
  Vehicle Base ID/1 -> Subtract/2
  Subtract/1 -> If/1
  If/1 -> Switch Case Action Subsystem2/Action

== system AdaptiveCruiseControl_HapticInterface/Can Network Inputs/Extract CAN data/Data to s,n,psi,us 3 ==
  Vehicle Base ID : Inport
  CAN ID : Inport  Port=2
  Data : Inport  Port=3
  If : If  IfExpression=u1 == 5  ElseIfExpressions=u1 == 6  ShowElse=off
  Mux3 : Mux
  Subtract : Sum  Inputs=+-
  Switch Case Action Subsystem2 : Subsystem  TreatAsAtomicUnit=on
  Switch Case Action Subsystem3 : Subsystem  TreatAsAtomicUnit=on
  Out1 : Outport  VectorParamsAs1DForOutWhenUnconnected=off
  wires:
  If/2 -> Switch Case Action Subsystem3/Action
  Switch Case Action Subsystem2/2(n) -> Mux3/2
  Mux3/1 -> Out1/1
  Switch Case Action Subsystem3/2(us) -> Mux3/4
  Switch Case Action Subsystem3/1(psi) -> Mux3/3
  Data/1 -> Switch Case Action Subsystem2/1(s,n), Switch Case Action Subsystem3/1(psi,us)
  Switch Case Action Subsystem2/1(s) -> Mux3/1
  CAN ID/1 -> Subtract/1
  Vehicle Base ID/1 -> Subtract/2
  Subtract/1 -> If/1
  If/1 -> Switch Case Action Subsystem2/Action

== system AdaptiveCruiseControl_HapticInterface/Can Network Inputs/Extract CAN data/Data to s,n,psi,us 4 ==
  Vehicle Base ID : Inport
  CAN ID : Inport  Port=2
  Data : Inport  Port=3
  If : If  IfExpression=u1 == 5  ElseIfExpressions=u1 == 6  ShowElse=off
  Mux3 : Mux
  Subtract : Sum  Inputs=+-
  Switch Case Action Subsystem2 : Subsystem  TreatAsAtomicUnit=on
  Switch Case Action Subsystem3 : Subsystem  TreatAsAtomicUnit=on
  Out1 : Outport  VectorParamsAs1DForOutWhenUnconnected=off
  wires:
  If/2 -> Switch Case Action Subsystem3/Action
  Switch Case Action Subsystem2/2(n) -> Mux3/2
  Mux3/1 -> Out1/1
  Switch Case Action Subsystem3/2(us) -> Mux3/4
  Switch Case Action Subsystem3/1(psi) -> Mux3/3
  Data/1 -> Switch Case Action Subsystem2/1(s,n), Switch Case Action Subsystem3/1(psi,us)
  Switch Case Action Subsystem2/1(s) -> Mux3/1
  CAN ID/1 -> Subtract/1
  Vehicle Base ID/1 -> Subtract/2
  Subtract/1 -> If/1
  If/1 -> Switch Case Action Subsystem2/Action

== system AdaptiveCruiseControl_HapticInterface/Can Network Inputs/Extract CAN data/Data to s,n,psi,us 5 ==
  Vehicle Base ID : Inport
  CAN ID : Inport  Port=2
  Data : Inport  Port=3
  If : If  IfExpression=u1 == 5  ElseIfExpressions=u1 == 6  ShowElse=off
  Mux3 : Mux
  Subtract : Sum  Inputs=+-
  Switch Case Action Subsystem2 : Subsystem  TreatAsAtomicUnit=on
  Switch Case Action Subsystem3 : Subsystem  TreatAsAtomicUnit=on
  Out1 : Outport  VectorParamsAs1DForOutWhenUnconnected=off
  wires:
  If/2 -> Switch Case Action Subsystem3/Action
  Switch Case Action Subsystem2/2(n) -> Mux3/2
  Mux3/1 -> Out1/1
  Switch Case Action Subsystem3/2(us) -> Mux3/4
  Switch Case Action Subsystem3/1(psi) -> Mux3/3
  Data/1 -> Switch Case Action Subsystem2/1(s,n), Switch Case Action Subsystem3/1(psi,us)
  Switch Case Action Subsystem2/1(s) -> Mux3/1
  CAN ID/1 -> Subtract/1
  Vehicle Base ID/1 -> Subtract/2
  Subtract/1 -> If/1
  If/1 -> Switch Case Action Subsystem2/Action

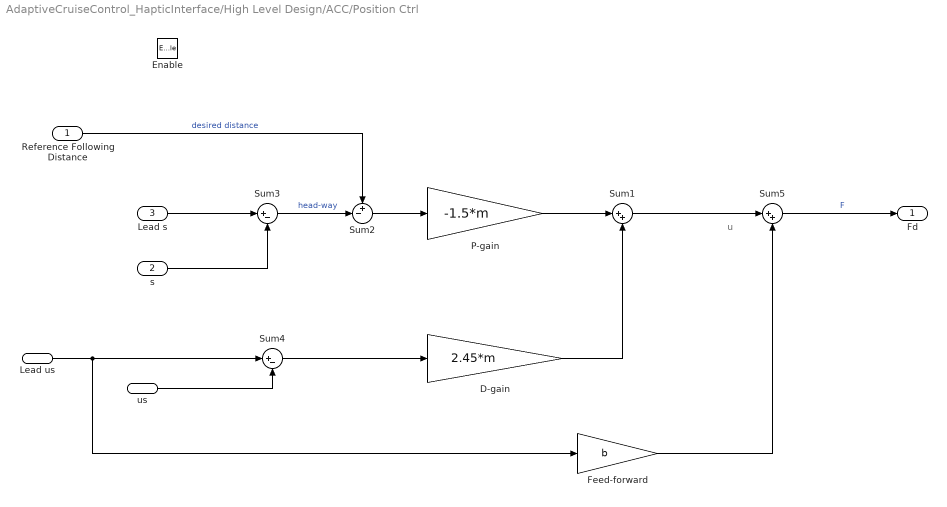
== system AdaptiveCruiseControl_HapticInterface/High Level Design/ACC/Position Ctrl ==
  note: u
  Reference Following Distance : Inport
  s : Inport  Port=2
  Lead s : Inport  Port=3
  us : Inport  Port=4
  Lead us : Inport  Port=5
  Enable : EnablePort
  D-gain : Gain  Gain=2.45*m  SaturateOnIntegerOverflow=on  OutDataTypeStr=Inherit: Same as input  ParamDataTypeStr=Inherit: Same as input
  Feed-forward : Gain  Gain=b  SaturateOnIntegerOverflow=on  OutDataTypeStr=Inherit: Same as input  ParamDataTypeStr=Inherit: Same as input
  P-gain : Gain  Gain=-1.5*m  SaturateOnIntegerOverflow=on  OutDataTypeStr=Inherit: Same as input  ParamDataTypeStr=Inherit: Same as input
  Sum1 : Sum  Inputs=|++  SaturateOnIntegerOverflow=on
  Sum2 : Sum  Inputs=+-|  SaturateOnIntegerOverflow=on
  Sum3 : Sum  Inputs=|+-  SaturateOnIntegerOverflow=on
  Sum4 : Sum  Inputs=|+-  SaturateOnIntegerOverflow=on
  Sum5 : Sum  Inputs=|++  OutDataTypeStr=single  SaturateOnIntegerOverflow=on
  Fd : Outport
  wires:
  Sum1/1 -> Sum5/1
  Sum5/1 -> Fd/1  "F"
  Feed-forward/1 -> Sum5/2
  Sum4/1 -> D-gain/1
  Lead us/1 -> Feed-forward/1, Sum4/1
  us/1 -> Sum4/2
  D-gain/1 -> Sum1/2
  P-gain/1 -> Sum1/1
  Sum2/1 -> P-gain/1
  Sum3/1 -> Sum2/2  "head-way"
  Reference Following Distance/1 -> Sum2/1  "desired distance"
  s/1 -> Sum3/2
  Lead s/1 -> Sum3/1

== system AdaptiveCruiseControl_HapticInterface/High Level Design/ACC/Speed Ctrl ==
  Speed Set Point : Inport
  Speed : Inport  Port=2
  Enable : EnablePort
  Gain : Gain  Gain=b  SaturateOnIntegerOverflow=on  OutDataTypeStr=Inherit: Same as input  ParamDataTypeStr=Inherit: Same as input
  PI : Subsystem
  Sum : Sum  Inputs=++|  OutDataTypeStr=single  SaturateOnIntegerOverflow=on
  Sum1 : Sum  Inputs=|+-  SaturateOnIntegerOverflow=on
  Fd : Outport
  wires:
  PI/1(U) -> Sum/2
  Gain/1 -> Sum/1
  Sum1/1 -> PI/1(Error)
  Speed/1 -> Sum1/2
  Speed Set Point/1 -> Sum1/1, Gain/1  "desired speed"
  Sum/1 -> Fd/1  "Fd"

== system AdaptiveCruiseControl_HapticInterface/High Level Design/ACC/Subsystem ==
  In1 : Inport
  Enable : EnablePort
  Out1 : Outport
  wires:
  In1/1 -> Out1/1

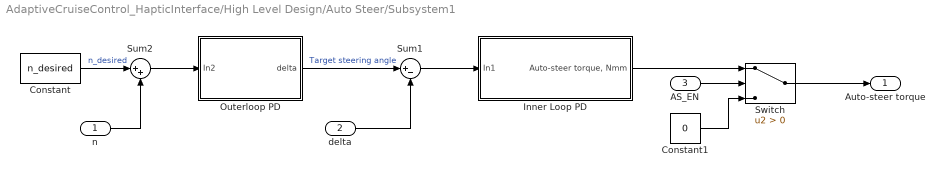
== system AdaptiveCruiseControl_HapticInterface/High Level Design/Auto Steer/Subsystem1 ==
  n : Inport
  delta : Inport  Port=2
  AS_EN : Inport  Port=3
  Constant : Constant  Value=n_desired
  Constant1 : Constant  Value=0
  Inner Loop PD : Subsystem
  Outerloop PD : Subsystem
  Sum1 : Sum  Inputs=|+-
  Sum2 : Sum  Inputs=|++
  Switch : Switch  Criteria=u2 > Threshold  SaturateOnIntegerOverflow=off  InputSameDT=off
  Auto-steer torque : Outport
  wires:
  Sum1/1 -> Inner Loop PD/1(In1)
  Sum2/1 -> Outerloop PD/1(In2)
  n/1 -> Sum2/2
  Constant/1 -> Sum2/1  "n_desired"
  delta/1 -> Sum1/2
  Outerloop PD/1(delta) -> Sum1/1  "Target steering angle"
  Inner Loop PD/1("Auto-steer torque, Nmm") -> Switch/1
  Switch/1 -> Auto-steer torque/1
  AS_EN/1 -> Switch/2
  Constant1/1 -> Switch/3

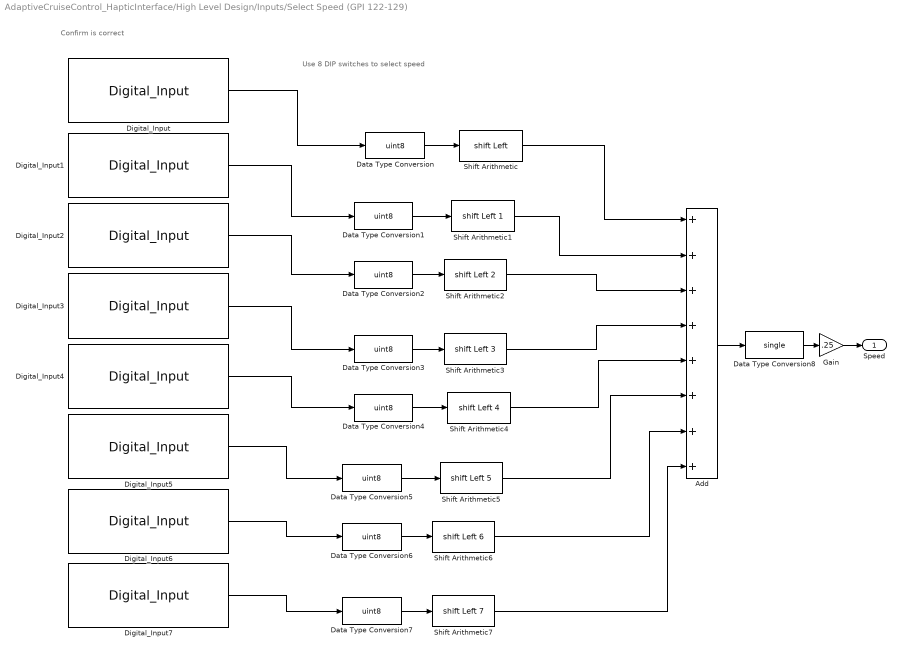
== system AdaptiveCruiseControl_HapticInterface/High Level Design/Inputs/Select Speed (GPI 122-129) ==
  note: Use 8 DIP switches to select speed
  note: Confirm is correct
  Add : Sum  Inputs=++++++++
  Data Type Conversion{,1..7} (8 alike) : DataTypeConversion  OutDataTypeStr=uint8  SaturateOnIntegerOverflow=off  RndMeth=Floor
  Data Type Conversion8 : DataTypeConversion  OutDataTypeStr=single  SaturateOnIntegerOverflow=off  RndMeth=Floor
  Digital_Input : mbd_s32k1xx_ec_toolbox/GPIO Blocks/Digital_Input  gpio_pin=PTE6: [PTE6 | Port E I/O]  pull_resistor=None  passive_filter=off
  Digital_Input1 : mbd_s32k1xx_ec_toolbox/GPIO Blocks/Digital_Input  gpio_pin=PTE7: [PTE7 | Port E I/O]  pull_resistor=None  passive_filter=off
  Digital_Input2 : mbd_s32k1xx_ec_toolbox/GPIO Blocks/Digital_Input  gpio_pin=PTE8: [PTE8 | Port E I/O]  pull_resistor=None  passive_filter=off
  Digital_Input3 : mbd_s32k1xx_ec_toolbox/GPIO Blocks/Digital_Input  gpio_pin=PTE9: [PTE9 | Port E I/O]  pull_resistor=None  passive_filter=off
  Digital_Input4 : mbd_s32k1xx_ec_toolbox/GPIO Blocks/Digital_Input  gpio_pin=PTE10: [PTE10 | Port E I/O]  pull_resistor=None  passive_filter=off
  Digital_Input5 : mbd_s32k1xx_ec_toolbox/GPIO Blocks/Digital_Input  gpio_pin=PTE11: [PTE11 | Port E I/O]  pull_resistor=None  passive_filter=off
  Digital_Input6 : mbd_s32k1xx_ec_toolbox/GPIO Blocks/Digital_Input  gpio_pin=PTE12: [PTE12 | Port E I/O]  pull_resistor=None  passive_filter=off
  Digital_Input7 : mbd_s32k1xx_ec_toolbox/GPIO Blocks/Digital_Input  gpio_pin=PTE13: [PTE13 | Port E I/O]  pull_resistor=None  passive_filter=off
  Gain : Gain  Gain=.25
  Shift Arithmetic : ArithShift  BitShiftDirection=Left
  Shift Arithmetic1 : ArithShift  BitShiftNumber=1  BitShiftDirection=Left
  Shift Arithmetic2 : ArithShift  BitShiftNumber=2  BitShiftDirection=Left
  Shift Arithmetic3 : ArithShift  BitShiftNumber=3  BitShiftDirection=Left
  Shift Arithmetic4 : ArithShift  BitShiftNumber=4  BitShiftDirection=Left
  Shift Arithmetic5 : ArithShift  BitShiftNumber=5  BitShiftDirection=Left
  Shift Arithmetic6 : ArithShift  BitShiftNumber=6  BitShiftDirection=Left
  Shift Arithmetic7 : ArithShift  BitShiftNumber=7  BitShiftDirection=Left
  Speed : Outport  VectorParamsAs1DForOutWhenUnconnected=off
  wires:
  Add/1 -> Data Type Conversion8/1
  Data Type Conversion8/1 -> Gain/1
  Gain/1 -> Speed/1
  Data Type Conversion1/1 -> Shift Arithmetic1/1
  Data Type Conversion3/1 -> Shift Arithmetic3/1
  Data Type Conversion/1 -> Shift Arithmetic/1
  Data Type Conversion2/1 -> Shift Arithmetic2/1
  Digital_Input/1 -> Data Type Conversion/1
  Digital_Input1/1 -> Data Type Conversion1/1
  Digital_Input2/1 -> Data Type Conversion2/1
  Digital_Input3/1 -> Data Type Conversion3/1
  Shift Arithmetic/1 -> Add/1
  Shift Arithmetic1/1 -> Add/2
  Shift Arithmetic2/1 -> Add/3
  Shift Arithmetic3/1 -> Add/4
  Data Type Conversion6/1 -> Shift Arithmetic6/1
  Data Type Conversion4/1 -> Shift Arithmetic4/1
  Data Type Conversion7/1 -> Shift Arithmetic7/1
  Data Type Conversion5/1 -> Shift Arithmetic5/1
  Digital_Input4/1 -> Data Type Conversion4/1
  Digital_Input5/1 -> Data Type Conversion5/1
  Digital_Input6/1 -> Data Type Conversion6/1
  Digital_Input7/1 -> Data Type Conversion7/1
  Shift Arithmetic4/1 -> Add/5
  Shift Arithmetic5/1 -> Add/6
  Shift Arithmetic6/1 -> Add/7
  Shift Arithmetic7/1 -> Add/8

== system AdaptiveCruiseControl_HapticInterface/High Level Design/Inputs/Throttle (Potentiometer) ==
  ADC_Start : mbd_s32k1xx_ec_toolbox/Motor Control Blocks/ADC Blocks/ADC_Start  instance=0  adc_r=A  adc_chan=PTA0: [ADC0_SE0 | ADC Single Ended Input]  aien=off  mcuTargetUpdate=on
  Constant : Constant  Value=pot_offset  OutDataTypeStr=single
  PotGain : Gain  Gain=pot_gain  OutDataTypeStr=single
  Sum : Sum  Inputs=|+-
  Fd : Outport  VectorParamsAs1DForOutWhenUnconnected=off
  wires:
  PotGain/1 -> Sum/1
  Constant/1 -> Sum/2
  Sum/1 -> Fd/1
  ADC_Start/1 -> PotGain/1

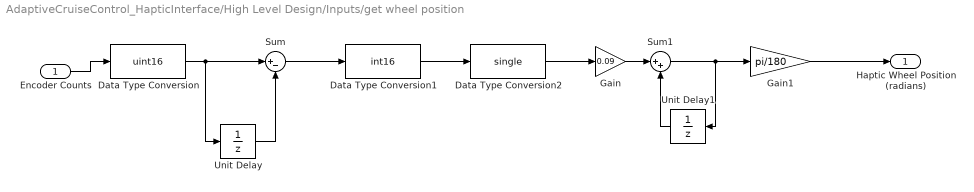
== system AdaptiveCruiseControl_HapticInterface/High Level Design/Inputs/get wheel position ==
  Encoder Counts : Inport
  Data Type Conversion : DataTypeConversion  OutDataTypeStr=uint16  SaturateOnIntegerOverflow=off  RndMeth=Floor
  Data Type Conversion1 : DataTypeConversion  OutDataTypeStr=int16  SaturateOnIntegerOverflow=off  RndMeth=Floor
  Data Type Conversion2 : DataTypeConversion  OutDataTypeStr=single  SaturateOnIntegerOverflow=off  RndMeth=Floor
  Gain : Gain  Gain=0.09
  Gain1 : Gain  Gain=pi/180
  Sum : Sum  Inputs=|+-
  Sum1 : Sum  Inputs=|++
  Unit Delay : UnitDelay  SampleTime=-1  HasFrameUpgradeWarning=on
  Unit Delay1 : UnitDelay  SampleTime=-1  HasFrameUpgradeWarning=on
  Haptic Wheel Position (radians) : Outport  VectorParamsAs1DForOutWhenUnconnected=off
  wires:
  Sum/1 -> Data Type Conversion1/1
  Unit Delay1/1 -> Sum1/2
  Data Type Conversion/1 -> Unit Delay/1, Sum/1
  Sum1/1 -> Gain1/1, Unit Delay1/1
  Unit Delay/1 -> Sum/2
  Data Type Conversion1/1 -> Data Type Conversion2/1
  Encoder Counts/1 -> Data Type Conversion/1
  Gain/1 -> Sum1/1
  Data Type Conversion2/1 -> Gain/1
  Gain1/1 -> Haptic Wheel Position (radians)/1

== system AdaptiveCruiseControl_HapticInterface/High Level Design/Outputs/Extract x,y,psi ==
  s,n,psi,us : Inport
  Demux : Demux
  Mux : Mux  Inputs=3
  Terminator : Terminator
  s,n to x,y : Veh_Sim/s,n to x,y  SystemSampleTime=-1  VariantActivationTime=update diagram  Latency=0  AutoFrameSizeCalculation=off
  x,y,psi : Outport  VectorParamsAs1DForOutWhenUnconnected=off
  wires:
  Demux/1 -> s,n to x,y/1
  Demux/2 -> s,n to x,y/2
  s,n,psi,us/1 -> Demux/1
  s,n to x,y/1 -> Mux/1
  s,n to x,y/2 -> Mux/2
  Demux/3 -> Mux/3
  Mux/1 -> x,y,psi/1
  Demux/4 -> Terminator/1

== system AdaptiveCruiseControl_HapticInterface/High Level Design/Outputs/Extract x,y,psi (Cars 1 - 6) ==
  s,n,psi,us (Cars 1 - 6) : Inport
  Demux : Demux  Outputs=6
  Extract x,y,psi : Subsystem
  Extract x,y,psi1 : Subsystem
  Extract x,y,psi2 : Subsystem
  Extract x,y,psi3 : Subsystem
  Extract x,y,psi4 : Subsystem
  Extract x,y,psi5 : Subsystem
  Mux : Mux  Inputs=6
  x,y,psi (Cars 1 - 6) : Outport  VectorParamsAs1DForOutWhenUnconnected=off
  wires:
  Demux/1 -> Extract x,y,psi/1(s,n,psi,us)
  Extract x,y,psi/1(x,y,psi) -> Mux/1
  Demux/2 -> Extract x,y,psi1/1(s,n,psi,us)
  Extract x,y,psi1/1(x,y,psi) -> Mux/2
  Demux/3 -> Extract x,y,psi2/1(s,n,psi,us)
  Extract x,y,psi2/1(x,y,psi) -> Mux/3
  Extract x,y,psi3/1(x,y,psi) -> Mux/4
  Demux/5 -> Extract x,y,psi4/1(s,n,psi,us)
  Extract x,y,psi4/1(x,y,psi) -> Mux/5
  s,n,psi,us (Cars 1 - 6)/1 -> Demux/1
  Extract x,y,psi5/1(x,y,psi) -> Mux/6
  Demux/6 -> Extract x,y,psi5/1(s,n,psi,us)
  Mux/1 -> x,y,psi (Cars 1 - 6)/1
  Demux/4 -> Extract x,y,psi3/1(s,n,psi,us)
